simulink model "solved_LQR_observer_R2016a"  (R2016a)
settings: Solver=ode45  StartTime=0.0  StopTime=simulation_time  MaxStep=0.01  RelTol=1e-3
undefined symbols (not defined in the file): AObs, BObs, C, CObs, Cprim, DObs, lqr_gain, LQR_input_signal_ID, parameters, path_to_track, sampling_time, x0, x0Obs
settings Model: Creator=ezequiel  LastModifiedBy=ezequiel
settings DebuggingCC: AllowSymbolicDim=off
settings ModelReferenceCC: PropagateSignalLabelsOutOfModel=off
settings GRTTargetCC: GeneratePreprocessorConditionals=Use local settings

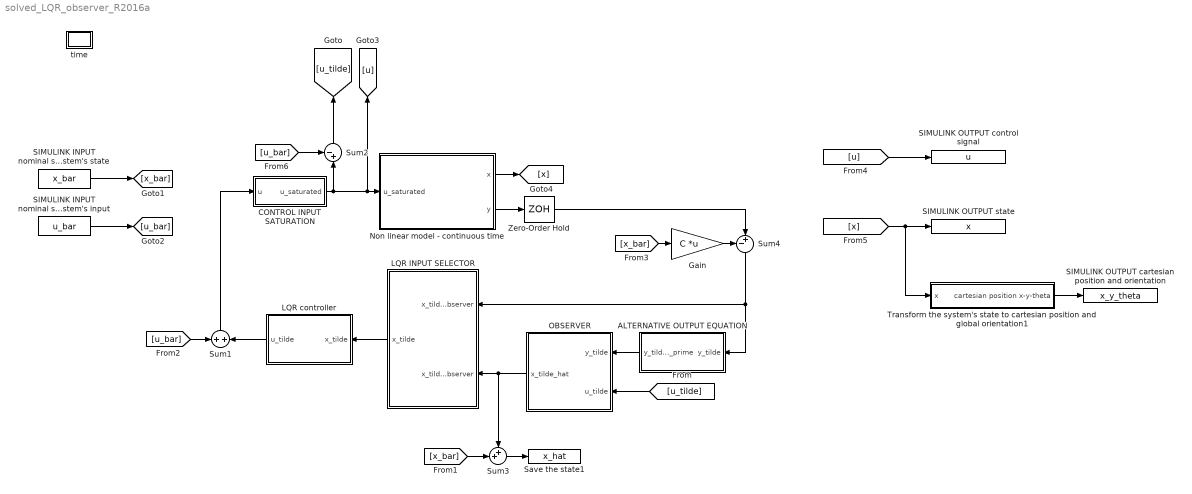
== system solved_LQR_observer_R2016a ==
  ALTERNATIVE OUTPUT EQUATION : Subsystem
  CONTROL INPUT SATURATION : Subsystem
  Gain : Gain  Gain=C  Multiplication=Matrix(K*u)
  LQR INPUT SELECTOR : Subsystem
  LQR controller : Subsystem
  Non linear model - continuous time : Subsystem
  OBSERVER : Subsystem
  SIMULINK INPUT nominal system's input : FromWorkspace  VariableName=u_bar  SampleTime=sampling_time  OutputAfterFinalValue=Holding final value
  SIMULINK INPUT nominal system's state : FromWorkspace  VariableName=x_bar  SampleTime=sampling_time  OutputAfterFinalValue=Holding final value
  SIMULINK OUTPUT cartesian position and orientation : ToWorkspace  VariableName=x_y_theta  SampleTime=-1
  SIMULINK OUTPUT control signal : ToWorkspace  VariableName=u  SampleTime=-1
  SIMULINK OUTPUT state : ToWorkspace  VariableName=x  SampleTime=-1
  Save the state1 : ToWorkspace  VariableName=x_hat  SampleTime=-1
  Sum1 : Sum  Inputs=+|+
  Sum2 : Sum  Inputs=-+|
  Sum3 : Sum  Inputs=++|
  Sum4 : Sum  Inputs=-+|
  Transform the system's state to cartesian position and global orientation1 : Subsystem
  Zero-Order Hold : ZeroOrderHold  SampleTime=sampling_time
  time : Subsystem
  wires:
  [u_bar] -> Sum1/1
  Non linear model - continuous time/2(y) -> Zero-Order Hold/1
  Sum2/1 -> [u_tilde]
  LQR controller/1(u_tilde) -> Sum1/2
  [x_bar] -> Gain/1
  Zero-Order Hold/1 -> Sum4/2
  Sum1/1 -> CONTROL INPUT SATURATION/1(u)
  Sum4/1 -> LQR INPUT SELECTOR/1("x_tilde_no_observer "), ALTERNATIVE OUTPUT EQUATION/1(y_tilde)
  Non linear model - continuous time/1(x) -> [x]
  [u_tilde] -> OBSERVER/2(u_tilde)
  CONTROL INPUT SATURATION/1(u_saturated) -> Non linear model - continuous time/1(u_saturated), [u], Sum2/2
  OBSERVER/1(x_tilde_hat) -> Sum3/1, LQR INPUT SELECTOR/2(x_tilde_observer)
  Gain/1 -> Sum4/1
  Sum3/1 -> Save the state1/1
  ALTERNATIVE OUTPUT EQUATION/1(y_tilde_prime) -> OBSERVER/1(y_tilde)
  LQR INPUT SELECTOR/1(x_tilde) -> LQR controller/1(x_tilde)
  [x_bar] -> Sum3/2
  SIMULINK INPUT nominal system's state/1 -> [x_bar]
  SIMULINK INPUT nominal system's input/1 -> [u_bar]
  [u] -> SIMULINK OUTPUT control signal/1
  [x] -> Transform the system's state to cartesian position and global orientation1/1(x), SIMULINK OUTPUT state/1
  Transform the system's state to cartesian position and global orientation1/1(cartesian position x-y-theta) -> SIMULINK OUTPUT cartesian position and orientation/1
  [u_bar] -> Sum2/1

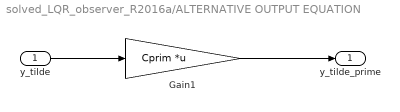
== system solved_LQR_observer_R2016a/ALTERNATIVE OUTPUT EQUATION ==
  y_tilde : Inport
  Gain1 : Gain  Gain=Cprim  Multiplication=Matrix(K*u)
  y_tilde_prime : Outport
  wires:
  y_tilde/1 -> Gain1/1
  Gain1/1 -> y_tilde_prime/1

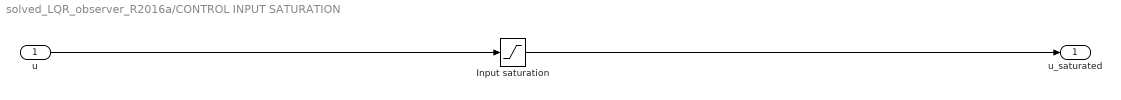
== system solved_LQR_observer_R2016a/CONTROL INPUT SATURATION ==
  u : Inport
  Input saturation : Saturate  UpperLimit=[Inf;4*pi]  LowerLimit=[0;-4*pi]
  u_saturated : Outport
  wires:
  u/1 -> Input saturation/1
  Input saturation/1 -> u_saturated/1

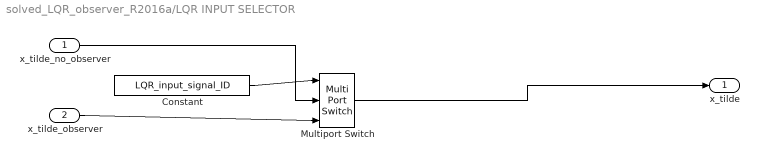
== system solved_LQR_observer_R2016a/LQR INPUT SELECTOR ==
  "x_tilde_no_observer " : Inport  PortDimensions=5
  x_tilde_observer : Inport  Port=2  PortDimensions=5
  Constant : Constant  Value=LQR_input_signal_ID
  Multiport Switch : MultiPortSwitch  Inputs=2
  x_tilde : Outport
  wires:
  "x_tilde_no_observer "/1 -> Multiport Switch/2
  x_tilde_observer/1 -> Multiport Switch/3
  Constant/1 -> Multiport Switch/1
  Multiport Switch/1 -> x_tilde/1

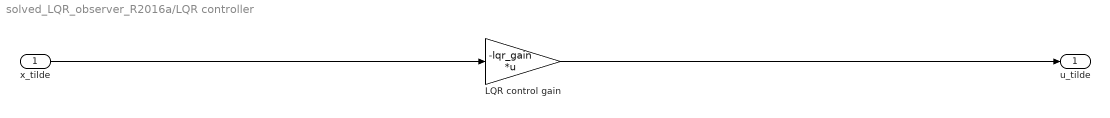
== system solved_LQR_observer_R2016a/LQR controller ==
  x_tilde : Inport  PortDimensions=5
  LQR control gain : Gain  Gain=-lqr_gain  Multiplication=Matrix(K*u)
  u_tilde : Outport
  wires:
  x_tilde/1 -> LQR control gain/1
  LQR control gain/1 -> u_tilde/1

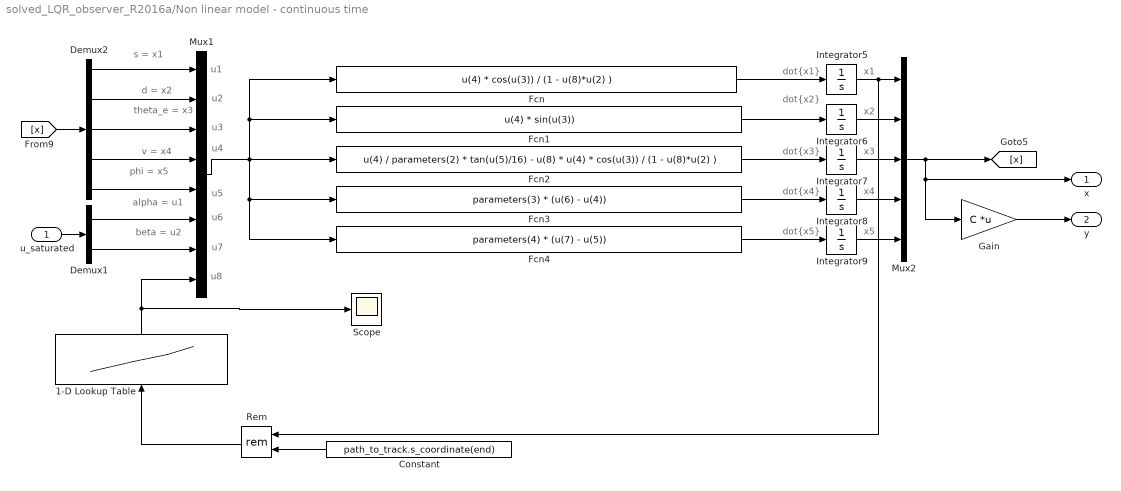
== system solved_LQR_observer_R2016a/Non linear model - continuous time ==
  note: s = x1
  note: dot{x1}
  note: d = x2
  note: theta_e = x3
  note: v = x4
  note: phi = x5
  note: alpha = u1
  note: beta = u2
  note: u1
  note: u2
  note: u3
  note: u4
  note: u5
  note: u6
  note: u7
  note: x1
  note: dot{x2}
  note: x2
  note: dot{x3}
  note: x3
  note: dot{x4}
  note: x4
  note: dot{x5}
  note: x5
  note: u8
  u_saturated : Inport
  1-D Lookup Table : Lookup_n-D  NumberOfTableDimensions=1  BreakpointsForDimension1=path_to_track.s_coordinate  Table=path_to_track.curvature  InternalRulePriority=Speed  RndMeth=Simplest  InputSameDT=on
  Constant : Constant  Value=path_to_track.s_coordinate(end)
  Demux1 : Demux  Outputs=2
  Demux2 : Demux  Outputs=5
  Fcn : Fcn  Expr=u(4) * cos(u(3)) / (1 - u(8)*u(2) )
  Fcn1 : Fcn  Expr=u(4) * sin(u(3))
  Fcn2 : Fcn  Expr=u(4) / parameters(2) * tan(u(5)/16) - u(8) * u(4) * cos(u(3)) / (1 - u(8)*u(2) )
  Fcn3 : Fcn  Expr=parameters(3) * (u(6) - u(4))
  Fcn4 : Fcn  Expr=parameters(4) * (u(7) - u(5))
  Gain : Gain  Gain=C  Multiplication=Matrix(K*u)
  Integrator5 : Integrator  InitialCondition=x0(1)
  Integrator6 : Integrator  InitialCondition=x0(2)
  Integrator7 : Integrator  InitialCondition=x0(3)
  Integrator8 : Integrator  InitialCondition=x0(4)
  Integrator9 : Integrator  InitialCondition=x0(5)
  Mux1 : Mux  Inputs=8
  Mux2 : Mux  Inputs=5
  Rem : Math  Operator=rem  SaturateOnIntegerOverflow=on
  Scope : Scope
  x : Outport
  y : Outport  Port=2
  wires:
  u_saturated/1 -> Demux1/1
  Fcn/1 -> Integrator5/1
  Demux2/1 -> Mux1/1
  Demux2/2 -> Mux1/2
  Demux2/3 -> Mux1/3
  Demux2/4 -> Mux1/4
  Demux2/5 -> Mux1/5
  Demux1/1 -> Mux1/6
  Demux1/2 -> Mux1/7
  Mux1/1 -> Fcn3/1, Fcn4/1, Fcn1/1, Fcn/1, Fcn2/1
  Fcn1/1 -> Integrator6/1
  Integrator6/1 -> Mux2/2
  Fcn2/1 -> Integrator7/1
  Integrator7/1 -> Mux2/3
  Fcn3/1 -> Integrator8/1
  Integrator8/1 -> Mux2/4
  Fcn4/1 -> Integrator9/1
  Integrator9/1 -> Mux2/5
  [x] -> Demux2/1
  1-D Lookup Table/1 -> Scope/1, Mux1/8
  Rem/1 -> 1-D Lookup Table/1
  Constant/1 -> Rem/2
  Integrator5/1 -> Rem/1, Mux2/1
  Mux2/1 -> Gain/1, x/1, [x]
  Gain/1 -> y/1

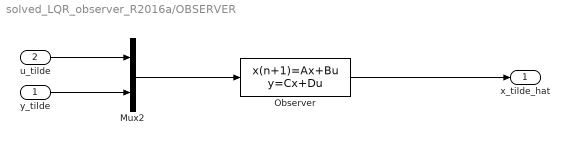
== system solved_LQR_observer_R2016a/OBSERVER ==
  y_tilde : Inport
  u_tilde : Inport  Port=2
  Mux2 : Mux  Inputs=2
  Observer : DiscreteStateSpace  A=AObs  B=BObs  C=CObs  D=DObs  X0=x0Obs  SampleTime=sampling_time
  x_tilde_hat : Outport
  wires:
  Mux2/1 -> Observer/1
  u_tilde/1 -> Mux2/1
  y_tilde/1 -> Mux2/2
  Observer/1 -> x_tilde_hat/1

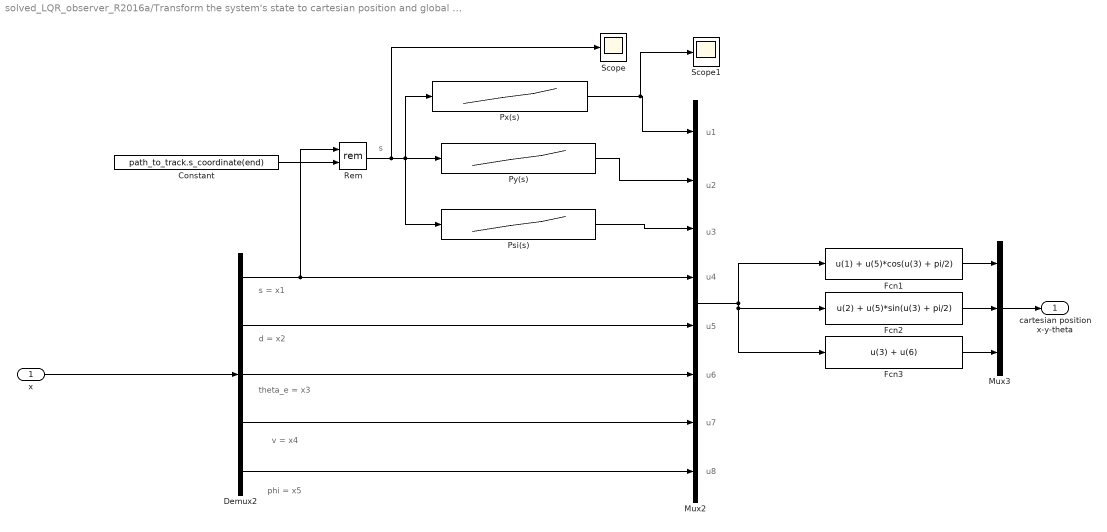
== system solved_LQR_observer_R2016a/Transform the system's state to cartesian position and global orientation1 ==
  note: s
  note: s = x1
  note: d = x2
  note: theta_e = x3
  note: v = x4
  note: phi = x5
  note: u1
  note: u2
  note: u3
  note: u4
  note: u5
  note: u6
  note: u7
  note: u8
  x : Inport
  Constant : Constant  Value=path_to_track.s_coordinate(end)
  Demux2 : Demux  Outputs=5
  Fcn1 : Fcn  Expr=u(1) + u(5)*cos(u(3) + pi/2)
  Fcn2 : Fcn  Expr=u(2) + u(5)*sin(u(3) + pi/2)
  Fcn3 : Fcn  Expr=u(3) + u(6)
  Mux2 : Mux  Inputs=8
  Mux3 : Mux  Inputs=3
  Psi(s) : Lookup_n-D  NumberOfTableDimensions=1  BreakpointsForDimension1=path_to_track.s_coordinate  Table=path_to_track.orientation  InternalRulePriority=Speed  RndMeth=Simplest  InputSameDT=on
  Px(s) : Lookup_n-D  NumberOfTableDimensions=1  BreakpointsForDimension1=path_to_track.s_coordinate  Table=path_to_track.coordinates(:,1)  InternalRulePriority=Speed  RndMeth=Simplest  InputSameDT=on
  Py(s) : Lookup_n-D  NumberOfTableDimensions=1  BreakpointsForDimension1=path_to_track.s_coordinate  Table=path_to_track.coordinates(:,2)  InternalRulePriority=Speed  RndMeth=Simplest  InputSameDT=on
  Rem : Math  Operator=rem  SaturateOnIntegerOverflow=on
  Scope : Scope
  Scope1 : Scope
  cartesian position x-y-theta : Outport
  wires:
  Demux2/1 -> Mux2/4, Rem/1
  Mux3/1 -> cartesian position x-y-theta/1
  x/1 -> Demux2/1
  Rem/1 -> Scope/1, Psi(s)/1, Px(s)/1, Py(s)/1
  Constant/1 -> Rem/2
  Px(s)/1 -> Scope1/1, Mux2/1
  Py(s)/1 -> Mux2/2
  Psi(s)/1 -> Mux2/3
  Mux2/1 -> Fcn3/1, Fcn2/1, Fcn1/1
  Fcn1/1 -> Mux3/1
  Fcn2/1 -> Mux3/2
  Fcn3/1 -> Mux3/3
  Demux2/2 -> Mux2/5
  Demux2/3 -> Mux2/6
  Demux2/4 -> Mux2/7
  Demux2/5 -> Mux2/8

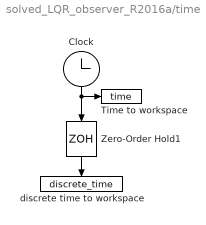
== system solved_LQR_observer_R2016a/time ==
  Clock : Clock
  Time to workspace : ToWorkspace  VariableName=time  SampleTime=-1
  Zero-Order Hold1 : ZeroOrderHold  SampleTime=sampling_time
  discrete time to workspace : ToWorkspace  VariableName=discrete_time  SampleTime=-1
  wires:
  Clock/1 -> Zero-Order Hold1/1, Time to workspace/1
  Zero-Order Hold1/1 -> discrete time to workspace/1
